simulink model "piCtrlCh6"  (R2014a)
settings: configuration reference "globalConfig" (kept outside this file)
undefined symbols (not defined in the file): gcbh, Ki, Kp, rmidispblock, Ts
settings Model: RequirementInfo={'other' 'throttleReqsCh6.doc' '@pi_ctrl_1' 'true' 'Must implement standard proportional plus integral control algorithm.' '' ; 'other' 'throttleReqsCh6.doc' '@pi_ctrl_2' 'true' 'Proportional and integral gains should be adjustable.' '' ; 'other' 'throttleReqsCh6.doc' '@pi_ctrl_3' 'true' 'Measures must be taken to prevent windup in integral state.' '' } %GIDa_8782a213_6690_4762_8fd4_78a65de31043  Creator=jrivitus  LastModifiedBy=scastro

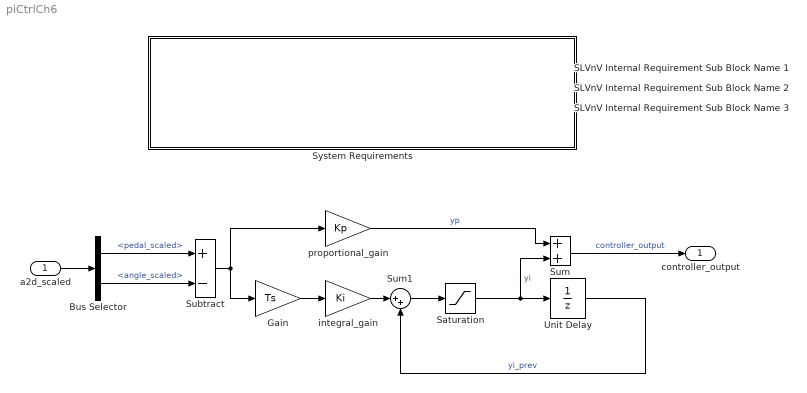
== system piCtrlCh6 ==
  a2d_scaled : Inport  OutDataTypeStr=Bus: a2d_scaled_bus  PortDimensions=1  SampleTime=Ts
  Bus Selector : BusSelector  OutputSignals=pedal_scaled,angle_scaled
  Gain : Gain  Gain=Ts  SaturateOnIntegerOverflow=on  OutDataTypeStr=Inherit: Same as input  ParamDataTypeStr=Inherit: Same as input
  SLVnV Internal Requirement Sub Block Name 1 : Subsystem  mask(System Requirement Item){label=0, index=1}
      mask init:
      | label = rmidispblock('label',index);
      settings: CopyFcn=rmidispblock('copyReq',gcbh)  DeleteFcn=rmidispblock('deleteReq',gcbh);  OpenFcn=rmidispblock('openReq',gcbh)  MoveFcn=rmidispblock('move',gcbh);
      mask Display: text(0,0,label,'horizontalAlignment','left','verticalAlignment','bottom')
  SLVnV Internal Requirement Sub Block Name 2 : Subsystem  mask(System Requirement Item){label=0, index=2}
      mask init:
      | label = rmidispblock('label',index);
      settings: CopyFcn=rmidispblock('copyReq',gcbh)  DeleteFcn=rmidispblock('deleteReq',gcbh);  OpenFcn=rmidispblock('openReq',gcbh)  MoveFcn=rmidispblock('move',gcbh);
      mask Display: text(0,0,label,'horizontalAlignment','left','verticalAlignment','bottom')
  SLVnV Internal Requirement Sub Block Name 3 : Subsystem  mask(System Requirement Item){label=0, index=3}
      mask init:
      | label = rmidispblock('label',index);
      settings: CopyFcn=rmidispblock('copyReq',gcbh)  DeleteFcn=rmidispblock('deleteReq',gcbh);  OpenFcn=rmidispblock('openReq',gcbh)  MoveFcn=rmidispblock('move',gcbh);
      mask Display: text(0,0,label,'horizontalAlignment','left','verticalAlignment','bottom')
  Saturation : Saturate  UpperLimit=1  LowerLimit=-1
      settings: AttributesFormatString=Max: %<UpperLimit>\nMin: %<LowerLimit>
  Subtract : Sum  Inputs=+-
  Sum : Sum  SaturateOnIntegerOverflow=on  InputSameDT=on  OutDataTypeStr=Inherit: Same as first input
  Sum1 : Sum  Inputs=|++  SaturateOnIntegerOverflow=on  InputSameDT=on  OutDataTypeStr=Inherit: Same as first input
  System Requirements : Subsystem  LoadFcn=rmidispblock('load',gcbh)  mask(System Requirements){id=SystemReq, title=System Requirements}
      mask prompts: title "Block Title"
      mask help: Lists the requirements for the current model.
      mask init:
      | id = 'SystemReq';
      | [w,h] = rmidispblock('display',gcbh);
      settings: CopyFcn=rmidispblock('create',gcbh)  DeleteFcn=rmidispblock('delete',gcbh)  ModelCloseFcn=rmidispblock('close',gcbh)  PreSaveFcn=rmidispblock('close',gcbh)  PostSaveFcn=rmidispblock('open',gcbh)  OpenFcn=rmidispblock('open',gcbh)  MoveFcn=rmidispblock('move',gcbh)
      mask Help: helpview(fullfile(docroot,'toolbox','slvnv','slvnv.map'),'systemrequirements')
      mask Display: text(424/2,109-4,rmidispblock('title',gcbh),'horizontalAlignment','center','verticalAlignment','top')
  Unit Delay : UnitDelay  SampleTime=Ts
      settings: AttributesFormatString=yi0 = %<X0>\nSample time = %<SampleTime>
  integral_gain : Gain  Gain=Ki  SaturateOnIntegerOverflow=on  OutDataTypeStr=Inherit: Same as input  ParamDataTypeStr=Inherit: Same as input
  proportional_gain : Gain  Gain=Kp  SaturateOnIntegerOverflow=on  OutDataTypeStr=Inherit: Same as input  ParamDataTypeStr=Inherit: Same as input
  controller_output : Outport  OutDataTypeStr=double  PortDimensions=1  SampleTime=Ts
  wires:
  a2d_scaled/1 -> Bus Selector/1
  Subtract/1 -> Gain/1, proportional_gain/1
  Bus Selector/2 -> Subtract/2  "<angle_scaled>"
  Bus Selector/1 -> Subtract/1  "<pedal_scaled>"
  proportional_gain/1 -> Sum/1  "yp"
  integral_gain/1 -> Sum1/1
  Gain/1 -> integral_gain/1
  Unit Delay/1 -> Sum1/2  "yi_prev"
  Sum1/1 -> Saturation/1
  Saturation/1 -> Unit Delay/1, Sum/2  "yi"
  Sum/1 -> controller_output/1  "controller_output"

== system piCtrlCh6/SLVnV Internal Requirement Sub Block Name 1 ==

== system piCtrlCh6/SLVnV Internal Requirement Sub Block Name 2 ==

== system piCtrlCh6/SLVnV Internal Requirement Sub Block Name 3 ==

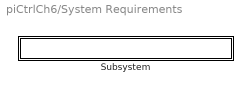
== system piCtrlCh6/System Requirements ==
  Subsystem : Subsystem  mask{label=0, index=1}
      mask init:
      | label = rmidispblock('label',index);
      settings: OpenFcn=rmidispblock('openReq',gcbh);
      mask Display: text(0,0,label,'horizontalAlignment','left','verticalAlignment','bottom')

== system piCtrlCh6/System Requirements/Subsystem ==
